simulink model "sl_fforwardTraj"  (R2014a)
settings: Solver=ode45  StartTime=0.0  StopTime=10.0  RelTol=1e-3
libraries: roblocks x3
settings Model: Creator=corkep  LastModifiedBy=timk
settings DataIOCC: SignalLoggingSaveFormat=ModelDataLogs
settings OptimizationCC: ExpressionDepthLimit=2147483647
settings DebuggingCC: UnderspecifiedInitializationDetection=Classic  FcnCallInpInsideContextMsg=UseLocalSettings  StateNameClashWarn=warning
settings GRTTargetCC: CombineOutputUpdateFcns=off  GRTInterface=on

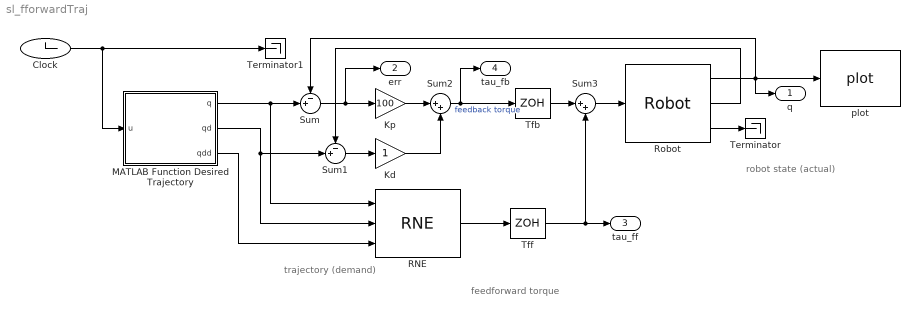
== system sl_fforwardTraj ==
  note: trajectory
      | (demand)
  note: robot state
      | (actual)
  note: feedforward torque
  Clock : Clock
  Kd : Gain  SaturateOnIntegerOverflow=on  OutDataTypeStr=Inherit: Same as input  ParamDataTypeStr=Inherit: Same as input
  Kp : Gain  Gain=100  SaturateOnIntegerOverflow=on  OutDataTypeStr=Inherit: Same as input  ParamDataTypeStr=Inherit: Same as input
  MATLAB Function Desired Trajectory : MATLAB Function  TreatAsAtomicUnit=on
  RNE : roblocks/Dynamics/RNE  robot=myRobot  grav=[0 0 9.81]
  Robot : roblocks/Dynamics/Robot  robot=myRobot  q0=[0 0 0 0 0 0]
  Sum : Sum  Inputs=-+|  SaturateOnIntegerOverflow=on  InputSameDT=on  OutDataTypeStr=Inherit: Same as first input
  Sum1 : Sum  Inputs=-+|  SaturateOnIntegerOverflow=on  InputSameDT=on  OutDataTypeStr=Inherit: Same as first input
  Sum2 : Sum  Inputs=|++  SaturateOnIntegerOverflow=on  InputSameDT=on  OutDataTypeStr=Inherit: Same as first input
  Sum3 : Sum  Inputs=|++  SaturateOnIntegerOverflow=on  InputSameDT=on  OutDataTypeStr=Inherit: Same as first input
  Terminator : Terminator
  Terminator1 : Terminator
  Tfb : ZeroOrderHold  SampleTime=0.01
  Tff : ZeroOrderHold  SampleTime=0.01
  plot : roblocks/Robot Graphics/plot  robot=myRobot  fps=25  holdplot=on
  q : Outport
  err : Outport  Port=2
  tau_ff : Outport  Port=3
  tau_fb : Outport  Port=4
  wires:
  Kd/1 -> Sum2/2
  Sum/1 -> Kp/1, err/1
  Kp/1 -> Sum2/1
  Sum1/1 -> Kd/1
  Sum2/1 -> Tfb/1, tau_fb/1  "feedback torque"
  Sum3/1 -> Robot/1
  Robot/1 -> plot/1, Sum/1, q/1
  Robot/2 -> Sum1/1
  MATLAB Function Desired Trajectory/1(q) -> RNE/1, Sum/2
  MATLAB Function Desired Trajectory/2(qd) -> Sum1/2, RNE/2
  MATLAB Function Desired Trajectory/3(qdd) -> RNE/3
  Robot/3 -> Terminator/1
  Tff/1 -> Sum3/2, tau_ff/1
  Tfb/1 -> Sum3/1
  RNE/1 -> Tff/1
  Clock/1 -> MATLAB Function Desired Trajectory/1(u), Terminator1/1

== matlab function sl_fforwardTraj/MATLAB Function Desired Trajectory ==
  data: u input; q output; qd output; qdd output
% Allows creation of a trajectory as a function of time.  All code 
% should be self-containted.  This will compiled by simulink into mex
%   input - time in sec
%   output - joint angle, velocity, and acceleration : q, qd, qdd
%
% writen by Tim K. for ME 8287. 2015
function [q,qd,qdd ] = desiredTrajectory(u)
%#codegen

t = u(1);  % sample time
A = 1;  % amplitude/circle radius
k = 1;  % speed


%               x                y        z | orientation
q   = [      A*sin(k*t)       A*cos(k*t)  0     0 0 0   ]'; 
qd  = [    k*A*cos(k*t)    -k*A*sin(k*t)  0     0 0 0   ]'; 
qdd = [ -k^2*A*sin(k*t)  -k^2*A*cos(k*t)  0     0 0 0   ]';
